simulink model "sasControl"  (R2020a)
settings: Solver=ode45  StartTime=0.0  StopTime=0.8  MaxStep=5e-06  RelTol=1e-9  AbsTol=4e-3
undefined symbols (not defined in the file): Asigma, b1, b2, bsigma, C, Csigma, CvC, Cxe, L, LiL, LoadAddResistor, LoadRemoveResistor, Masigma, Nasigma, obsControl, obsSys, P, R, Ro, SourceAddVoltage, SourceRemoveVoltage, taua1, taua2, Tmax, Vin, x0, x_e, xe
libraries: powerlib x36, PhdLibrary x8, dspsigops x3, powerlib_meascontrol x2
settings Model: SimulationMode=accelerator  Creator=d13go  LastModifiedBy=d13go
settings SolverCC: ZeroCrossControl=DisableAll  ZeroCrossAlgorithm=Adaptive
settings DebuggingCC: IgnoredZcDiagnostic=none

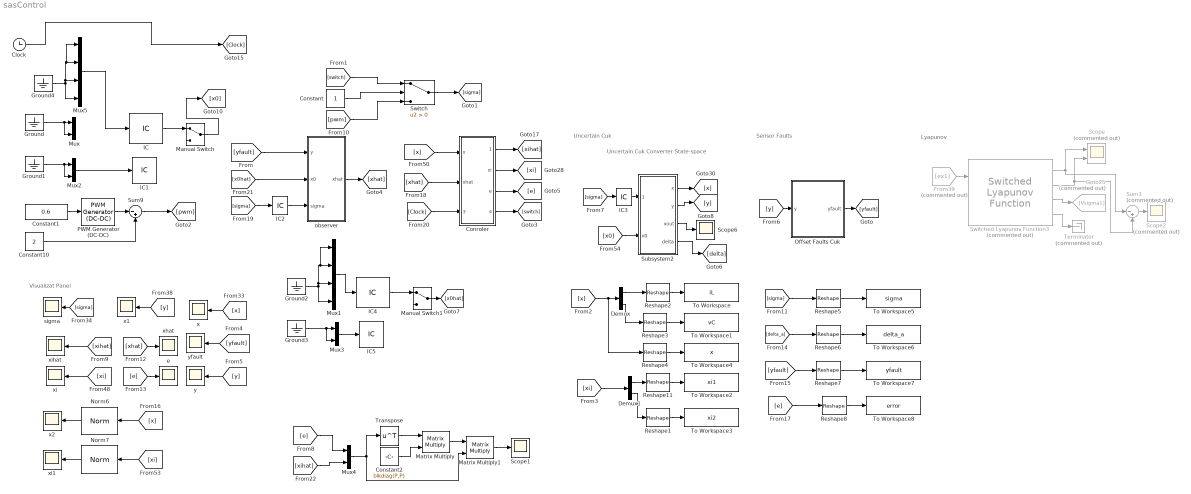
== system sasControl ==
  note: Visualizat Panel
  note: Sensor Faults
  note: Uncertain Cuk Converter
      | State-space
  note: Uncertain Cuk
  note: Lyapunov
  Clock : Clock
  Conroler : Subsystem
  Constant : Constant
  Constant1 : Constant  Value=0.6
  Constant10 : Constant  Value=2
  Constant2 : Constant  Value=blkdiag(P,P)
  Demux : Demux  Outputs=2
  Demux1 : Demux  Outputs=2
  From39 : From  Commented=on  GotoTag=ex1
  Goto25 : Goto  Commented=on  GotoTag=Vsigma1
  Ground{,1..4} (5 alike) : Ground
  IC : InitialCondition  Value=[x0]
  IC1 : InitialCondition  Value=[0 0]
  IC2 : InitialCondition  Value=2
  IC3 : InitialCondition  Value=2
  IC4 : InitialCondition  Value=[x0]
  IC5 : InitialCondition  Value=[0 0]
  Manual Switch : ManualSwitch
  Manual Switch1 : ManualSwitch
  Matrix Multiply : Product  Multiplication=Matrix(*)
  Matrix Multiply1 : Product  Multiplication=Matrix(*)
  Mux{,2..4} (4 alike) : Mux  Inputs=2
  Mux1 : Mux
  Mux5 : Mux
  Norm6 : PhdLibrary/Norms/Norm
      settings: SourceProductName=Phd Diego
  Norm7 : PhdLibrary/Norms/Norm
      settings: SourceProductName=Phd Diego
  Offset Faults Cuk : Subsystem
  PWM Generator (DC-DC) : powerlib_meascontrol/Pulse & Signal Generators/PWM Generator (DC-DC)  Fsw=10000  Ts=5e-6
  Reshape{1..8,11} (9 alike) : Reshape
  Scope : Scope  Commented=on  NumInputPorts=2
  Scope1 : Scope
  Scope2 : Scope  Commented=on
  Scope6 : Scope
  Subsystem2 : Subsystem
  Sum3 : Sum  Commented=on  Inputs=|-+
  Sum9 : Sum  Inputs=|-+
  Switch : Switch  Criteria=u2 > Threshold
  Switched Lyapunov Function3 : PhdLibrary/Switched Lyapunov Function  Commented=on  P1=obsSys{1}.lmiMat.P{1}  P2=obsSys{1}.lmiMat.P{2}
      link override Quadratic Lyapunov Function2: SourceBlock=PhdLibrary/Quadratic Lyapunov Function
      link override Quadratic Lyapunov Function3: SourceBlock=PhdLibrary/Quadratic Lyapunov Function
      settings: SourceProductName=Phd Diego
  Terminator : Terminator  Commented=on
  To Workspace : ToWorkspace  VariableName=iL  SaveFormat=Timeseries  SampleTime=-1
  To Workspace1 : ToWorkspace  VariableName=vC  SaveFormat=Timeseries  SampleTime=-1
  To Workspace2 : ToWorkspace  VariableName=xi1  SaveFormat=Timeseries  SampleTime=-1
  To Workspace3 : ToWorkspace  VariableName=xi2  SaveFormat=Timeseries  SampleTime=-1
  To Workspace4 : ToWorkspace  VariableName=x  SaveFormat=Timeseries  SampleTime=-1
  To Workspace5 : ToWorkspace  VariableName=sigma  SaveFormat=Timeseries  SampleTime=-1
  To Workspace6 : ToWorkspace  VariableName=delta_a  SaveFormat=Timeseries  SampleTime=-1
  To Workspace7 : ToWorkspace  VariableName=yfault  SaveFormat=Timeseries  SampleTime=-1
  To Workspace8 : ToWorkspace  VariableName=error  SaveFormat=Timeseries  SampleTime=-1
  Transpose : Math  Operator=transpose  SaturateOnIntegerOverflow=on
  e : Scope
  observer : Subsystem
  sigma : Scope
  x : Scope
  x1 : Scope
  x2 : Scope
  xhat : Scope
  xi : Scope
  xi1 : Scope
  xihat : Scope
  y : Scope
  yfault : Scope
  wires:
  Subsystem2/1(x) -> [x]
  Subsystem2/2(y) -> [y]
  [y] -> Offset Faults Cuk/1(y)
  Offset Faults Cuk/1(yfault) -> [yfault]
  [yfault] -> observer/1(y)
  [sigma] -> IC3/1
  [x] -> x/1
  [sigma] -> sigma/1
  [y] -> x1/1
  From39/1 -> Switched Lyapunov Function3/1
  Switched Lyapunov Function3/3 -> Goto25/1
  Switched Lyapunov Function3/4 -> Terminator/1
  Switched Lyapunov Function3/1 -> Scope/1, Sum3/1
  Switched Lyapunov Function3/2 -> Sum3/2, Scope/2
  Conroler/1(xihat) -> [xihat]
  [xihat] -> xihat/1
  [xi] -> xi/1
  Sum3/1 -> Scope2/1
  PWM Generator (DC-DC)/1 -> Sum9/1
  Constant10/1 -> Sum9/2
  Constant1/1 -> PWM Generator (DC-DC)/1
  Conroler/2(xi) -> [xi]
  [x0] -> Subsystem2/2(x0)
  Ground/1 -> Mux/2, Mux/1
  [x] -> Reshape4/1, Demux/1
  Demux/1 -> Reshape2/1
  Demux/2 -> Reshape3/1
  [xi] -> Demux1/1
  Demux1/1 -> Reshape11/1
  Reshape11/1 -> To Workspace2/1
  Reshape1/1 -> To Workspace3/1
  Demux1/2 -> Reshape1/1
  Norm7/1 -> xi1/1
  [x] -> Norm6/1
  [xi] -> Norm7/1
  Norm6/1 -> x2/1
  [yfault] -> yfault/1
  [y] -> y/1
  Ground1/1 -> Mux2/2, Mux2/1
  Mux2/1 -> IC1/1
  [x0hat] -> observer/2(x0)
  Subsystem2/3(xout) -> Scope6/1
  IC/1 -> Manual Switch/1
  Manual Switch/1 -> [x0]
  Sum9/1 -> [pwm]
  observer/1(xhat) -> [xhat]
  Conroler/3(e) -> [e]
  [xhat] -> xhat/1
  [e] -> e/1
  Reshape2/1 -> To Workspace/1
  Reshape3/1 -> To Workspace1/1
  Reshape4/1 -> To Workspace4/1
  Conroler/4(sigma) -> [switch]
  [switch] -> Switch/1
  [pwm] -> Switch/3
  Constant/1 -> Switch/2
  Switch/1 -> [sigma]
  [sigma] -> Reshape5/1
  Reshape5/1 -> To Workspace5/1
  Subsystem2/4(delta) -> [delta]
  [delta_a] -> Reshape6/1
  Reshape6/1 -> To Workspace6/1
  Reshape7/1 -> To Workspace7/1
  [yfault] -> Reshape7/1
  [e] -> Reshape8/1
  Reshape8/1 -> To Workspace8/1
  [Clock] -> Conroler/3(clock)
  [x] -> Conroler/1(x)
  [sigma] -> IC2/1
  IC2/1 -> observer/3(sigma)
  IC3/1 -> Subsystem2/1(sigma)
  [xhat] -> Conroler/2(xhat)
  Mux1/1 -> IC4/1
  Ground2/1 -> Mux1/1, Mux1/2, Mux1/3, Mux1/4
  Mux3/1 -> IC5/1
  Ground3/1 -> Mux3/2, Mux3/1
  Manual Switch1/1 -> [x0hat]
  IC4/1 -> Manual Switch1/1
  [e] -> Mux4/1
  [xihat] -> Mux4/2
  Mux4/1 -> Matrix Multiply1/2, Transpose/1
  Matrix Multiply/1 -> Matrix Multiply1/1
  Matrix Multiply1/1 -> Scope1/1
  Constant2/1 -> Matrix Multiply/2
  Transpose/1 -> Matrix Multiply/1
  Mux5/1 -> IC/1
  Ground4/1 -> Mux5/1, Mux5/2, Mux5/3, Mux5/4
  Clock/1 -> [Clock]

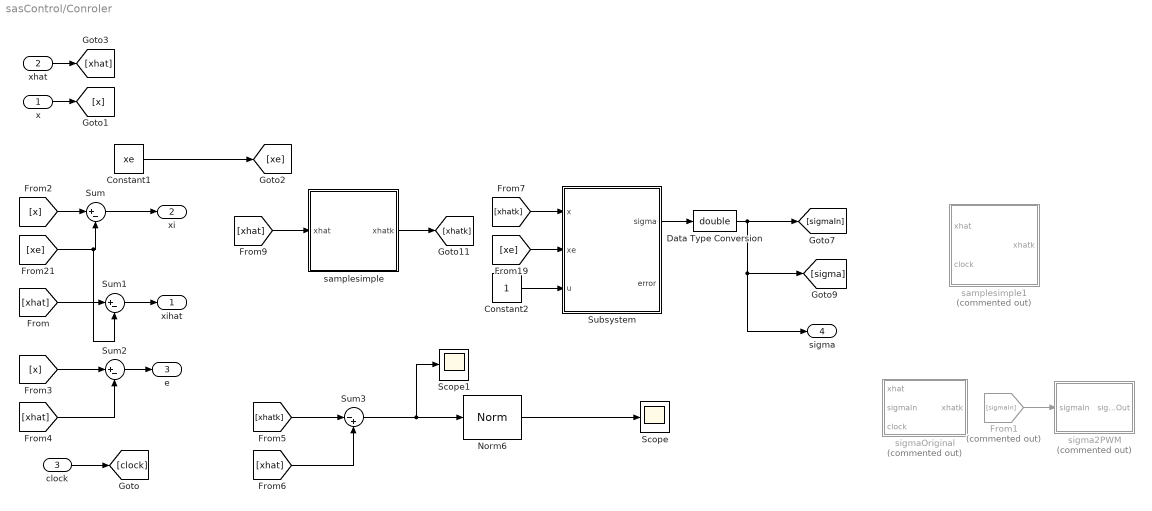
== system sasControl/Conroler ==
  x : Inport
  xhat : Inport  Port=2
  clock : Inport  Port=3
  Constant1 : Constant  Value=xe  VectorParams1D=off
  Constant2 : Constant
  Data Type Conversion : DataTypeConversion  OutDataTypeStr=double
  From1 : From  Commented=on  GotoTag=sigmaIn
  Norm6 : PhdLibrary/Norms/Norm
      settings: SourceProductName=Phd Diego
  Scope : Scope
  Scope1 : Scope
  Subsystem : Subsystem  mask{P1=obsControl.P, A1=obsControl.Asigma{1}, B1=obsControl.bsigma{1}, P2=obsControl.P, A2=obsControl.Asigma{2}, B2=obsControl.bsigma{2}}
      mask prompts: P1 "P matrx"; A1 "A matrix"; B1 "b matrix"; P2 "P matrx"; A2 "A matrix"; B2 "b matrix"
      mask DialogControl Container3 Prompt: Subsystem 1
      mask DialogControl Container3_copy Prompt: Subsystem 2
      mask Display: disp('Switching \n Control Law \n 2-Subsystems');
  Sum : Sum  Inputs=|+-
  Sum1 : Sum  Inputs=|+-
  Sum2 : Sum  Inputs=|+-
  Sum3 : Sum  Inputs=|-+
  samplesimple : Subsystem
  samplesimple1 : Subsystem  Commented=on
  sigma2PWM : Subsystem  Commented=on
  sigmaOriginal : Subsystem  Commented=on
  xihat : Outport
  xi : Outport  Port=2
  e : Outport  Port=3
  sigma : Outport  Port=4
  wires:
  [xe] -> Sum1/2, Sum/2
  xhat/1 -> [xhat]
  x/1 -> [x]
  Sum2/1 -> e/1
  samplesimple/1("xhatk ") -> [xhatk]
  Sum1/1 -> xihat/1
  [xe] -> Subsystem/2(xe)
  Constant2/1 -> Subsystem/3(u)
  Subsystem/1(sigma) -> Data Type Conversion/1
  Data Type Conversion/1 -> sigma/1, [sigma], [sigmaIn]
  From1/1 -> sigma2PWM/1(sigmaIn)
  clock/1 -> [clock]
  Sum/1 -> xi/1
  Constant1/1 -> [xe]
  [xhat] -> Sum1/1
  [x] -> Sum/1
  [x] -> Sum2/1
  [xhat] -> Sum2/2
  [xhatk] -> Sum3/1
  Sum3/1 -> Scope1/1, Norm6/1
  [xhat] -> Sum3/2
  Norm6/1 -> Scope/1
  [xhat] -> samplesimple/1(xhat)
  [xhatk] -> Subsystem/1(x)

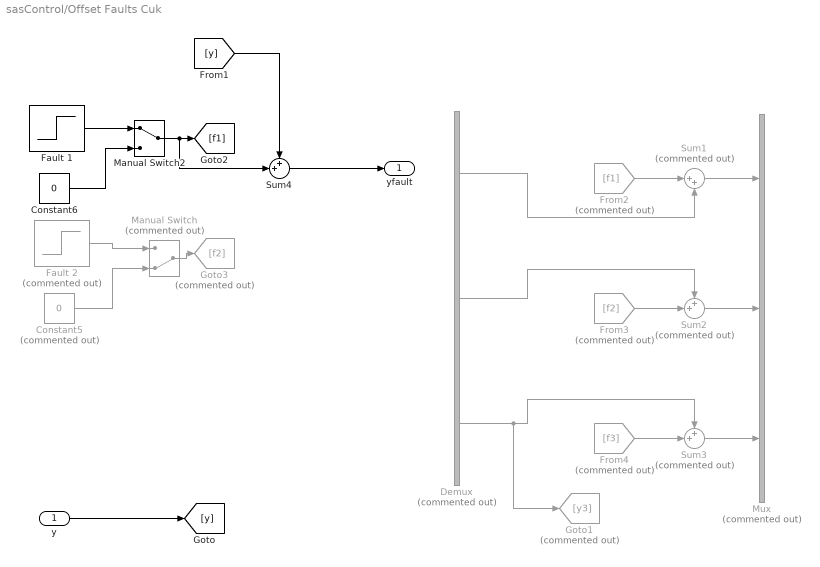
== system sasControl/Offset Faults Cuk ==
  y : Inport
  Constant5 : Constant  Commented=on  Value=0
  Constant6 : Constant  Value=0
  Demux : Demux  Commented=on  Outputs=3
  Fault 1 : Step  Time=0.35  After=0.5/7*Cxe(1)  SampleTime=0
  Fault 2 : Step  Commented=on  Time=0.35  After=0.075*Cxe(2)  SampleTime=0
  From2 : From  Commented=on  GotoTag=f1
  From3 : From  Commented=on  GotoTag=f2
  From4 : From  Commented=on  GotoTag=f3
  Goto1 : Goto  Commented=on  GotoTag=y3
  Goto3 : Goto  Commented=on  GotoTag=f2
  Manual Switch : ManualSwitch  Commented=on  CurrentSetting=0
  Manual Switch2 : ManualSwitch
  Mux : Mux  Commented=on  Inputs=3
  Sum1 : Sum  Commented=on  Inputs=|++
  Sum2 : Sum  Commented=on  Inputs=++|
  Sum3 : Sum  Commented=on  Inputs=++|
  Sum4 : Sum  Inputs=++|
  yfault : Outport
  wires:
  Fault 2/1 -> Manual Switch/1
  Fault 1/1 -> Manual Switch2/1
  Constant5/1 -> Manual Switch/2
  Constant6/1 -> Manual Switch2/2
  Sum1/1 -> Mux/1
  Sum3/1 -> Mux/3
  y/1 -> [y]
  Sum2/1 -> Mux/2
  Manual Switch2/1 -> Sum4/2, [f1]
  From2/1 -> Sum1/1
  Manual Switch/1 -> Goto3/1
  From3/1 -> Sum2/2
  From4/1 -> Sum3/2
  Demux/1 -> Sum1/2
  Demux/2 -> Sum2/1
  Demux/3 -> Goto1/1, Sum3/1
  [y] -> Sum4/1
  Sum4/1 -> yfault/1

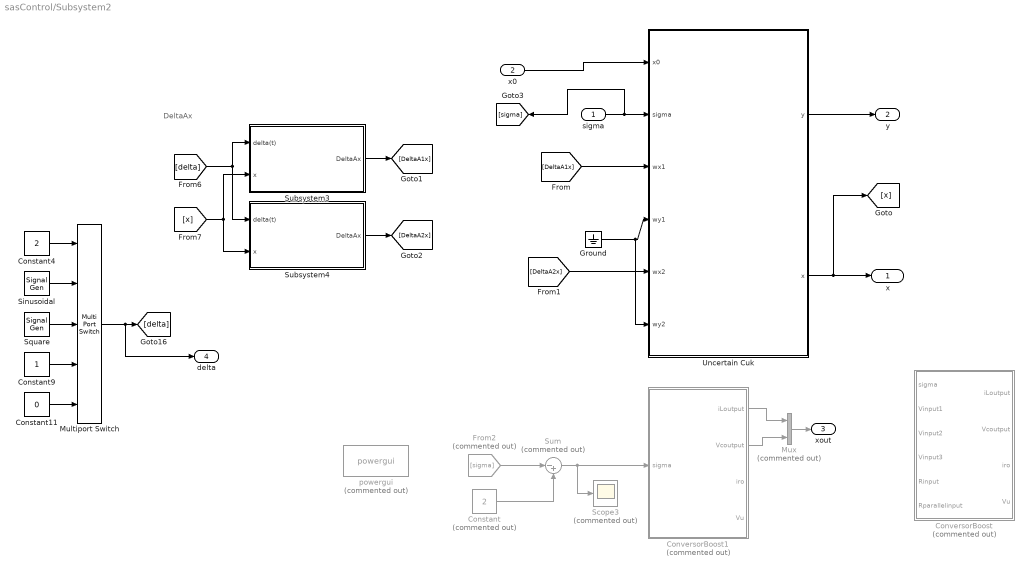
== system sasControl/Subsystem2 ==
  note: DeltaAx
  sigma : Inport
  x0 : Inport  Port=2
  Constant : Constant  Commented=on  Value=2
  Constant11 : Constant  Value=0
  Constant4 : Constant  Value=2
  Constant9 : Constant
  ConversorBoost : Subsystem  Commented=on
  ConversorBoost1 : Subsystem  Commented=on
  From2 : From  Commented=on  GotoTag=sigma
  Ground : Ground
  Multiport Switch : MultiPortSwitch  Inputs=4
  Mux : Mux  Commented=on  Inputs=2
  Scope3 : Scope  Commented=on
  Sinusoidal : SignalGenerator  Amplitude=20  Frequency=60  Units=rad/sec
  Square : SignalGenerator  WaveForm=square  Frequency=300  Units=rad/sec
  Subsystem3 : Subsystem  mask{M=Masigma{1}, N=Nasigma{1}}
      mask prompts: M "M matrix"; N "N matrix"
      mask DialogControl DescTextVar Prompt: Uncertainties matrices of type \DeltaA = delta(t)*MaNa*x(t)
      mask Display: disp('Norm-bounded \n uncertainty')
  Subsystem4 : Subsystem  mask{M=Masigma{2}, N=Nasigma{2}}
      mask prompts: M "M matrix"; N "N matrix"
      mask DialogControl DescTextVar Prompt: Uncertainties matrices of type \DeltaA = delta(t)*MaNa*x(t)
      mask Display: disp('Norm-bounded \n uncertainty')
  Sum : Sum  Commented=on  Inputs=|-+
  Uncertain Cuk : Subsystem  mask{A1=Asigma{1}, B1=bsigma{1}, C1=Csigma{1}, A2=Asigma{2}, B2=bsigma{2}, C2=Csigma{2}}
      mask prompts: A1 "Matrix A"; B1 "Matrix B"; C1 "Matrix C"; A2 "Matrix A"; B2 "Matrix B"; C2 "Matrix C"
      mask DialogControl DescTextVar Prompt: dx/dt = A(sigma)x+ B(sigma)u + wx(sigma,x,u,t)
      mask DialogControl Control2 Prompt: y = C(sigma)x + wy(sigma,x,u,t)
      mask DialogControl Container3 Prompt: Subsystem 1
      mask DialogControl Container4 Prompt: Subsystem 2
      mask Display: disp('Switched Perturbed State Space \n 2-Subsystems')
  powergui : powerlib/powergui  Priority=1  Commented=on  SimulationMode=Continuous  SampleTime=50e-6  frequency=60  Iterations=50  frequencyindice=0  Pbase=100e6  ErrMax=1e-4  UnitsV=kV  UnitsW=MW  buscounter=0  FunctionMessages=off  echomessages=off  EnableUseOfTLC=off  CurrentSourceSwitches=off  DisableSnubberDevices=off  DisableRonSwitches=off  DisableVfSwitches=off  DisplayEquations=off  AutomaticDiscreteSolvers=off  SolverType=Tustin/Backward Euler (TBE)  Interpol=off  ExternalGateDelay=off  methode=off  Ts=100  x0status=blocks  SPID=on  SwTol=0  HookPort=off  NonlinearTolerance=1e-4  nMaxIteration=100  ContinueOnMaxIteration=off  RestoreLinks=warning  ResistiveCurrentMeasurement=off  Frange=[0:2:500]  Ylog=off  Xlog=on  ShowGrid=off  save=off  variable=ZData  structure=0  ZoomFFT=off  StartTime=0.0  cycles=1  DisplayStyle=1  fundamental=60  FreqAxis=off  MaxFrequency=1000  frequencyindicesteady=1  RmsSteady=1  display=off
  x : Outport
  y : Outport  Port=2
  xout : Outport  Port=3
  delta : Outport  Port=4
  wires:
  x0/1 -> Uncertain Cuk/1(x0)
  Uncertain Cuk/2(x) -> [x], x/1
  Uncertain Cuk/1(y) -> y/1
  sigma/1 -> [sigma], Uncertain Cuk/2(sigma)
  [DeltaA1x] -> Uncertain Cuk/3(wx1)
  Constant9/1 -> Multiport Switch/4
  Sinusoidal/1 -> Multiport Switch/2
  Constant4/1 -> Multiport Switch/1
  Square/1 -> Multiport Switch/3
  Constant11/1 -> Multiport Switch/5
  [DeltaA2x] -> Uncertain Cuk/5(wx2)
  Multiport Switch/1 -> delta/1, [delta]
  Subsystem3/1(DeltaAx) -> [DeltaA1x]
  [x] -> Subsystem4/2(x), Subsystem3/2(x)
  [delta] -> Subsystem3/1(delta(t)), Subsystem4/1(delta(t))
  Ground/1 -> Uncertain Cuk/6(wy2), Uncertain Cuk/4(wy1)
  Subsystem4/1(DeltaAx) -> [DeltaA2x]
  ConversorBoost1/1(iLoutput) -> Mux/1
  ConversorBoost1/2(Vcoutput) -> Mux/2
  Mux/1 -> xout/1
  From2/1 -> Sum/1
  Sum/1 -> Scope3/1, ConversorBoost1/1(sigma)
  Constant/1 -> Sum/2

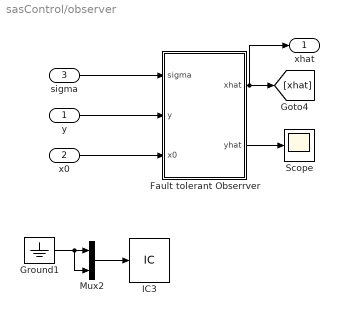
== system sasControl/observer ==
  y : Inport
  x0 : Inport  Port=2
  sigma : Inport  Port=3
  Fault tolerant Obserrver : Subsystem  mask(Boots State-Space model){A1=obsControl.Asigma{1,1}, A2=obsControl.Asigma{1,2}, B1=obsControl.bsigma{1,1}, Cmatrix=obsControl.Csigma{1,1}, L1=10*obsControl.Lcsigma{1,1}, L2=10*obsControl.Lcsigma{1,2}}
      mask prompts: A1 "A1 matrix"; A2 "A2 matrix"; B1 "B matrix"; Cmatrix "Output Matrix"; L1 "L1 matrix"; L2 "L2 matrix"
      mask help: Boots State-Space model
      mask Display: disp('Observer')
  Ground1 : Ground
  IC3 : InitialCondition  Value=[51 151]
  Mux2 : Mux  Inputs=2
  Scope : Scope
  xhat : Outport
  wires:
  Fault tolerant Obserrver/2(yhat) -> Scope/1
  y/1 -> Fault tolerant Obserrver/2(y)
  Fault tolerant Obserrver/1(xhat) -> xhat/1, [xhat]
  sigma/1 -> Fault tolerant Obserrver/1(sigma)
  Ground1/1 -> Mux2/2, Mux2/1
  Mux2/1 -> IC3/1
  x0/1 -> Fault tolerant Obserrver/3(x0)

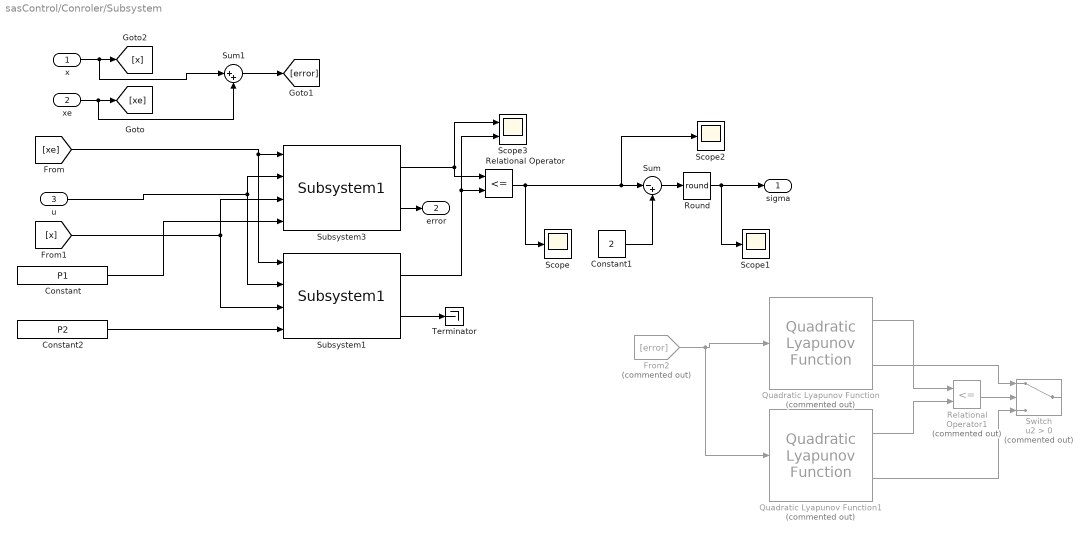
== system sasControl/Conroler/Subsystem ==
  x : Inport
  xe : Inport  Port=2
  u : Inport  Port=3
  Constant : Constant  Value=P1
  Constant1 : Constant  Value=2
  Constant2 : Constant  Value=P2
  From2 : From  Commented=on  GotoTag=error
  Quadratic Lyapunov Function : PhdLibrary/Quadratic Lyapunov Function  Commented=on  P=P1
      settings: SourceProductName=Phd Diego
  Quadratic Lyapunov Function1 : PhdLibrary/Quadratic Lyapunov Function  Commented=on  P=P2
      settings: SourceProductName=Phd Diego
  Relational Operator : RelationalOperator  Operator=<=  OutDataTypeStr=boolean  RndMeth=Nearest
  Relational Operator1 : RelationalOperator  Commented=on  Operator=<=  OutDataTypeStr=boolean  RndMeth=Nearest
  Round : Rounding  Operator=round
  Scope : Scope
  Scope1 : Scope
  Scope2 : Scope
  Scope3 : Scope  NumInputPorts=2
  Subsystem1 : PhdLibrary/Controllers/Subsystem1  A=A2  B=B2
      settings: SourceProductName=Phd Diego
  Subsystem3 : PhdLibrary/Controllers/Subsystem1  A=A1  B=B1
      settings: SourceProductName=Phd Diego
  Sum : Sum  Inputs=|-+
  Sum1 : Sum  Inputs=|++
  Switch : Switch  Commented=on  Criteria=u2 > Threshold
  Terminator : Terminator
  sigma : Outport
  error : Outport  Port=2
  wires:
  x/1 -> Sum1/1, [x]
  [xe] -> Subsystem1/1, Subsystem3/1
  [x] -> Subsystem1/3, Subsystem3/3
  u/1 -> Subsystem1/2, Subsystem3/2
  Subsystem1/2 -> Terminator/1
  Subsystem3/2 -> error/1
  Subsystem1/1 -> Scope3/2, Relational Operator/2
  Subsystem3/1 -> Relational Operator/1, Scope3/1
  Relational Operator/1 -> Scope2/1, Sum/1, Scope/1
  Constant1/1 -> Sum/2
  Sum/1 -> Round/1
  Round/1 -> Scope1/1, sigma/1
  xe/1 -> [xe], Sum1/2
  Sum1/1 -> [error]
  From2/1 -> Quadratic Lyapunov Function1/1, Quadratic Lyapunov Function/1
  Quadratic Lyapunov Function1/1 -> Relational Operator1/2
  Relational Operator1/1 -> Switch/2
  Quadratic Lyapunov Function1/2 -> Switch/3
  Quadratic Lyapunov Function/1 -> Relational Operator1/1
  Quadratic Lyapunov Function/2 -> Switch/1
  Constant/1 -> Subsystem3/4
  Constant2/1 -> Subsystem1/4

== system sasControl/Conroler/samplesimple ==
  xhat : Inport
  NOT : Logic  Operator=NOT  IconShape=distinctive  AllPortsSameDT=off  OutDataTypeStr=boolean
  Pulse Generator : DiscretePulseGenerator  PulseType=Time based  Period=2*10e-6  PulseWidth=50
  Sample and Hold : dspsigops/Sample and Hold  trig=Either edge  initCond=1  latchinput=off
  Scope : Scope
  "xhatk " : Outport
  wires:
  xhat/1 -> Sample and Hold/1
  Sample and Hold/1 -> Scope/1, "xhatk "/1
  Pulse Generator/1 -> NOT/1
  NOT/1 -> Sample and Hold/Trigger

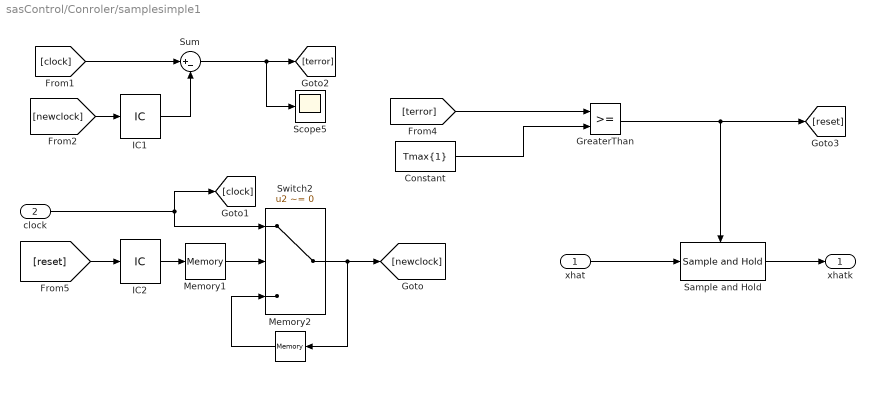
== system sasControl/Conroler/samplesimple1 ==
  xhat : Inport
  clock : Inport  Port=2
  Constant : Constant  Value=Tmax{1}
  GreaterThan : RelationalOperator  OutDataTypeStr=boolean  RndMeth=Simplest
  IC1 : InitialCondition  Value=0
  IC2 : InitialCondition  Value=0
  Memory1 : Memory  InheritSampleTime=on
  Memory2 : Memory  InheritSampleTime=on
  Sample and Hold : dspsigops/Sample and Hold  trig=Rising edge  initCond=1  latchinput=off
  Scope5 : Scope
  Sum : Sum  Inputs=|+-
  Switch2 : Switch  Criteria=u2 ~= 0
  "xhatk " : Outport
  wires:
  xhat/1 -> Sample and Hold/1
  Sample and Hold/1 -> "xhatk "/1
  [clock] -> Sum/1
  Sum/1 -> Scope5/1, [terror]
  Constant/1 -> GreaterThan/2
  [terror] -> GreaterThan/1
  GreaterThan/1 -> [reset], Sample and Hold/Trigger
  clock/1 -> [clock], Switch2/1
  [newclock] -> IC1/1
  IC1/1 -> Sum/2
  Switch2/1 -> [newclock], Memory2/1
  Memory2/1 -> Switch2/3
  [reset] -> IC2/1
  Memory1/1 -> Switch2/2
  IC2/1 -> Memory1/1

== system sasControl/Conroler/sigma2PWM ==
  sigmaIn : Inport
  Constant1 : Constant
  Constant10 : Constant  Value=2
  Constant3 : Constant  Value=0
  PWM Generator (DC-DC) : powerlib_meascontrol/Pulse & Signal Generators/PWM Generator (DC-DC)  Fsw=1  Ts=5e-6
  Sum9 : Sum  Inputs=|-+
  Switch1 : Switch  Threshold=2
  sigmaOut : Outport
  wires:
  Switch1/1 -> PWM Generator (DC-DC)/1
  PWM Generator (DC-DC)/1 -> Sum9/1
  Constant3/1 -> Switch1/1
  sigmaIn/1 -> Switch1/2
  Constant10/1 -> Sum9/2
  Sum9/1 -> sigmaOut/1
  Constant1/1 -> Switch1/3

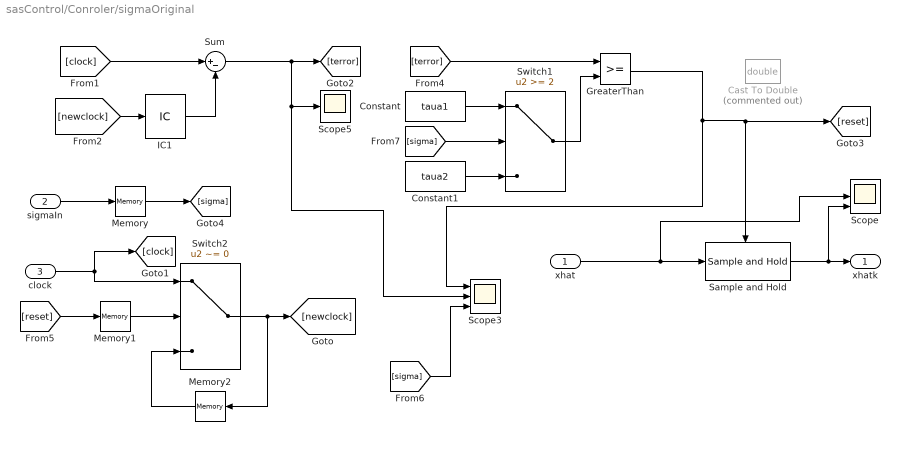
== system sasControl/Conroler/sigmaOriginal ==
  xhat : Inport
  sigmaIn : Inport  Port=2
  clock : Inport  Port=3
  Cast To Double : DataTypeConversion  Commented=on  OutDataTypeStr=double
  Constant : Constant  Value=taua1
  Constant1 : Constant  Value=taua2
  GreaterThan : RelationalOperator  OutDataTypeStr=boolean  RndMeth=Simplest
  IC1 : InitialCondition  Value=0
  Memory : Memory  InitialCondition=2  InheritSampleTime=on
  Memory1 : Memory  InitialCondition=2  InheritSampleTime=on
  Memory2 : Memory  InheritSampleTime=on
  Sample and Hold : dspsigops/Sample and Hold  trig=Rising edge  initCond=1  latchinput=off
  Scope : Scope  NumInputPorts=3
  Scope3 : Scope  NumInputPorts=3
  Scope5 : Scope
  Sum : Sum  Inputs=|+-
  Switch1 : Switch  Threshold=2
  Switch2 : Switch  Criteria=u2 ~= 0
  "xhatk " : Outport
  wires:
  xhat/1 -> Scope/2, Sample and Hold/1
  Sample and Hold/1 -> Scope/3, "xhatk "/1
  [clock] -> Sum/1
  Sum/1 -> Scope3/2, Scope5/1, [terror]
  Constant/1 -> Switch1/1
  Constant1/1 -> Switch1/3
  [terror] -> GreaterThan/1
  Switch1/1 -> GreaterThan/2
  GreaterThan/1 -> [reset], Sample and Hold/Trigger, Scope3/1
  clock/1 -> [clock], Switch2/1
  [reset] -> Memory1/1
  Memory1/1 -> Switch2/2
  [newclock] -> IC1/1
  IC1/1 -> Sum/2
  [sigma] -> Scope3/3
  Switch2/1 -> Memory2/1, [newclock]
  Memory2/1 -> Switch2/3
  [sigma] -> Switch1/2
  sigmaIn/1 -> Memory/1
  Memory/1 -> [sigma]

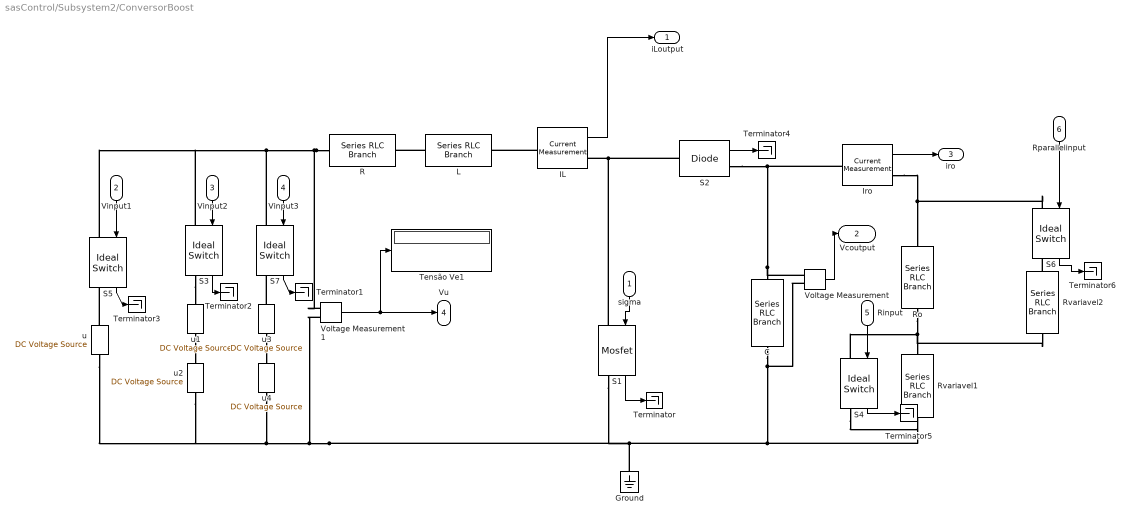
== system sasControl/Subsystem2/ConversorBoost ==
  sigma : Inport
  Vinput1 : Inport  Port=2
  Vinput2 : Inport  Port=3
  Vinput3 : Inport  Port=4
  Rinput : Inport  Port=5
  Rparallelinput : Inport  Port=6
  C : powerlib/Elements/Series RLC Branch  LConnTagsString=__new0  RConnTagsString=__new0  BranchType=C  Resistance=1  Inductance=1e-3  SetiL0=off  InitialCurrent=0  Capacitance=C  Setx0=on  InitialVoltage=0  Measurements=None
  Ground : powerlib/Elements/Ground  LConnTagsString=a
  IL : powerlib/Measurements/Current Measurement  PhasorSimulation=off  OutputType=Complex  PSBequivalent=0
  Iro : powerlib/Measurements/Current Measurement  PhasorSimulation=off  OutputType=Complex  PSBequivalent=0
  L : powerlib/Elements/Series RLC Branch  LConnTagsString=__new0  RConnTagsString=__new0  BranchType=L  Resistance=1  Inductance=L  SetiL0=on  InitialCurrent=0  Capacitance=1e-6  Setx0=off  InitialVoltage=0  Measurements=None
  R : powerlib/Elements/Series RLC Branch  LConnTagsString=__new0  RConnTagsString=__new0  BranchType=R  Resistance=R  Inductance=1e-3  SetiL0=off  InitialCurrent=0  Capacitance=1e-6  Setx0=off  InitialVoltage=0  Measurements=None
  Ro : powerlib/Elements/Series RLC Branch  LConnTagsString=__new0  RConnTagsString=__new0  BranchType=R  Resistance=Ro  Inductance=1e-3  SetiL0=off  InitialCurrent=0  Capacitance=1e-6  Setx0=off  InitialVoltage=0  Measurements=None
  Rvariavel1 : powerlib/Elements/Series RLC Branch  LConnTagsString=__new0  RConnTagsString=__new0  BranchType=R  Resistance=LoadAddResistor  Inductance=1e-3  SetiL0=off  InitialCurrent=0  Capacitance=1e-6  Setx0=off  InitialVoltage=0  Measurements=None
  Rvariavel2 : powerlib/Elements/Series RLC Branch  LConnTagsString=__new0  RConnTagsString=__new0  BranchType=R  Resistance=LoadRemoveResistor  Inductance=1e-3  SetiL0=off  InitialCurrent=0  Capacitance=1e-6  Setx0=off  InitialVoltage=0  Measurements=None
  S1 : powerlib/Power Electronics/Mosfet  Ron=0.0000001  Lon=0  Rd=0.000000001  Vfd=0  IC=0  Rs=1e5  Cs=inf  Measurements=on
  S2 : powerlib/Power Electronics/Diode  Ron=0.000001  Lon=0  Vf=0  IC=0  UseSnubber=off  Rs=0  Cs=0  Measurements=on
  S{3..7} (5 alike) : powerlib/Power Electronics/Ideal Switch  Ron=0.0000001  Lon=0  IC=0  Rs=1e8  Cs=inf  Measurements=on
  Tensão Ve1 : Display
  Terminator{,1..6} (7 alike) : Terminator
  Voltage Measurement : powerlib/Measurements/Voltage Measurement  PhasorSimulation=off  OutputType=Complex  PSBequivalent=0
  Voltage Measurement1 : powerlib/Measurements/Voltage Measurement  PhasorSimulation=off  OutputType=Complex  PSBequivalent=0
  u : powerlib/Electrical Sources/DC Voltage Source  Amplitude=u  Measurements=None
  u1 : powerlib/Electrical Sources/DC Voltage Source  Amplitude=SourceAddVoltage  Measurements=None
  u2 : powerlib/Electrical Sources/DC Voltage Source  Amplitude=u  Measurements=None
  u3 : powerlib/Electrical Sources/DC Voltage Source  Amplitude=SourceRemoveVoltage  Measurements=None
  u4 : powerlib/Electrical Sources/DC Voltage Source  Amplitude=u  Measurements=None
  iLoutput : Outport
  Vcoutput : Outport  Port=2
  iro : Outport  Port=3
  Vu : Outport  Port=4
  wires:
  Rinput/1 -> S4/1
  IL/1 -> iLoutput/1
  sigma/1 -> S1/1
  Voltage Measurement/1 -> Vcoutput/1
  Iro/1 -> iro/1
  Voltage Measurement1/1 -> Vu/1, Tensão Ve1/1
  Vinput1/1 -> S5/1
  Vinput2/1 -> S3/1
  Rparallelinput/1 -> S6/1
  Vinput3/1 -> S7/1
  S1/1 -> Terminator/1
  S7/1 -> Terminator1/1
  S3/1 -> Terminator2/1
  S5/1 -> Terminator3/1
  S2/1 -> Terminator4/1
  S4/1 -> Terminator5/1
  S6/1 -> Terminator6/1
  connections:
  Ro/RConn1 -- Rvariavel2/LConn1 -- Rvariavel1/RConn1 -- S4/LConn1
  IL/LConn1 -- L/RConn1
  C/RConn1 -- S4/RConn1 -- Rvariavel1/LConn1 -- S1/RConn1 -- u2/LConn1 -- u/LConn1 -- u4/LConn1 -- Voltage Measurement1/LConn2 -- Ground/LConn1 -- Voltage Measurement/LConn2
  S2/LConn1 -- S1/LConn1 -- IL/RConn1
  R/LConn1 -- S3/LConn1 -- S5/LConn1 -- S7/LConn1 -- Voltage Measurement1/LConn1
  Iro/RConn1 -- S6/LConn1 -- Ro/LConn1
  L/LConn1 -- R/RConn1
  S2/RConn1 -- Iro/LConn1 -- Voltage Measurement/LConn1 -- C/LConn1
  u/RConn1 -- S5/RConn1
  Rvariavel2/RConn1 -- S6/RConn1
  S3/RConn1 -- u1/RConn1
  u1/LConn1 -- u2/RConn1
  u3/LConn1 -- S7/RConn1
  u3/RConn1 -- u4/RConn1

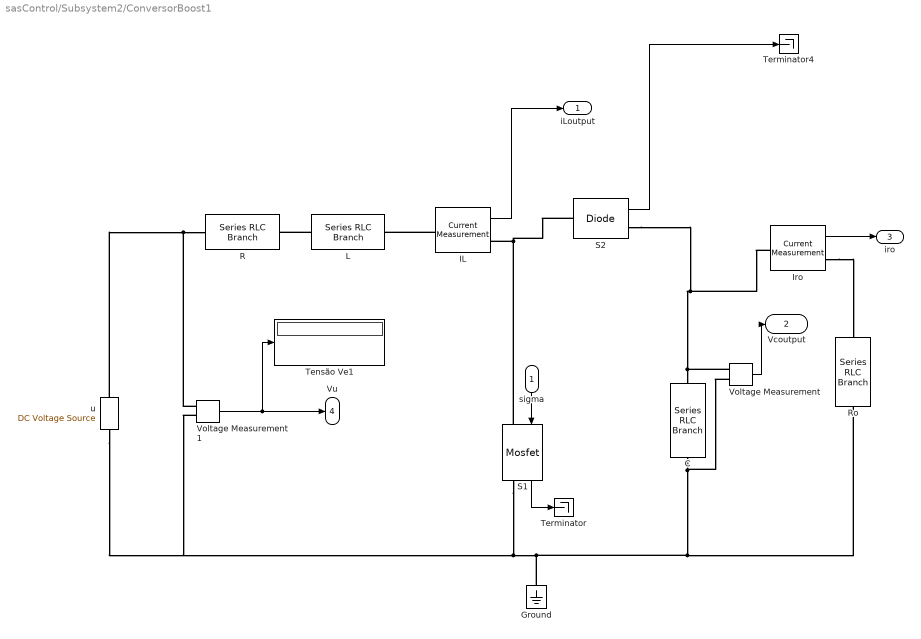
== system sasControl/Subsystem2/ConversorBoost1 ==
  sigma : Inport
  C : powerlib/Elements/Series RLC Branch  LConnTagsString=__new0  RConnTagsString=__new0  BranchType=C  Resistance=1  Inductance=1e-3  SetiL0=off  InitialCurrent=0  Capacitance=CvC  Setx0=on  InitialVoltage=xe(2)  Measurements=None
  Ground : powerlib/Elements/Ground  LConnTagsString=a
  IL : powerlib/Measurements/Current Measurement  PhasorSimulation=off  OutputType=Complex  PSBequivalent=0
  Iro : powerlib/Measurements/Current Measurement  PhasorSimulation=off  OutputType=Complex  PSBequivalent=0
  L : powerlib/Elements/Series RLC Branch  LConnTagsString=__new0  RConnTagsString=__new0  BranchType=L  Resistance=1  Inductance=LiL  SetiL0=on  InitialCurrent=0  Capacitance=1e-6  Setx0=off  InitialVoltage=0  Measurements=None
  R : powerlib/Elements/Series RLC Branch  LConnTagsString=__new0  RConnTagsString=__new0  BranchType=R  Resistance=R  Inductance=1e-3  SetiL0=off  InitialCurrent=0  Capacitance=1e-6  Setx0=off  InitialVoltage=0  Measurements=None
  Ro : powerlib/Elements/Series RLC Branch  LConnTagsString=__new0  RConnTagsString=__new0  BranchType=R  Resistance=Ro  Inductance=1e-3  SetiL0=off  InitialCurrent=0  Capacitance=1e-6  Setx0=off  InitialVoltage=0  Measurements=None
  S1 : powerlib/Power Electronics/Mosfet  Ron=0.0000001  Lon=0  Rd=0.000000001  Vfd=0  IC=0  Rs=1e5  Cs=inf  Measurements=on
  S2 : powerlib/Power Electronics/Diode  Ron=0.000001  Lon=0  Vf=0  IC=0  UseSnubber=off  Rs=0  Cs=0  Measurements=on
  Tensão Ve1 : Display
  Terminator : Terminator
  Terminator4 : Terminator
  Voltage Measurement : powerlib/Measurements/Voltage Measurement  PhasorSimulation=off  OutputType=Complex  PSBequivalent=0
  Voltage Measurement1 : powerlib/Measurements/Voltage Measurement  PhasorSimulation=off  OutputType=Complex  PSBequivalent=0
  u : powerlib/Electrical Sources/DC Voltage Source  Amplitude=Vin  Measurements=None
  iLoutput : Outport
  Vcoutput : Outport  Port=2
  iro : Outport  Port=3
  Vu : Outport  Port=4
  wires:
  IL/1 -> iLoutput/1
  sigma/1 -> S1/1
  Voltage Measurement/1 -> Vcoutput/1
  Iro/1 -> iro/1
  Voltage Measurement1/1 -> Vu/1, Tensão Ve1/1
  S1/1 -> Terminator/1
  S2/1 -> Terminator4/1
  connections:
  C/RConn1 -- Voltage Measurement/LConn2 -- Ro/RConn1 -- u/LConn1 -- Voltage Measurement1/LConn2 -- S1/RConn1 -- Ground/LConn1
  IL/LConn1 -- L/RConn1
  Voltage Measurement1/LConn1 -- u/RConn1 -- R/LConn1
  Iro/RConn1 -- Ro/LConn1
  L/LConn1 -- R/RConn1
  Iro/LConn1 -- S2/RConn1 -- Voltage Measurement/LConn1 -- C/LConn1
  S1/LConn1 -- S2/LConn1 -- IL/RConn1

== system sasControl/Subsystem2/Subsystem3 ==
  delta(t) : Inport
  x : Inport  Port=2
  Constant : Constant  Value=M
  Constant1 : Constant  Value=N
  Matrix Multiply1 : Product
  Matrix Multiply2 : Product  Multiplication=Matrix(*)
  Matrix Multiply3 : Product  Multiplication=Matrix(*)
  DeltaAx : Outport
  wires:
  Constant/1 -> Matrix Multiply3/1
  Constant1/1 -> Matrix Multiply3/2
  Matrix Multiply3/1 -> Matrix Multiply1/2
  delta(t)/1 -> Matrix Multiply1/1
  Matrix Multiply1/1 -> Matrix Multiply2/1
  x/1 -> Matrix Multiply2/2
  Matrix Multiply2/1 -> DeltaAx/1

== system sasControl/Subsystem2/Subsystem4 ==
  delta(t) : Inport
  x : Inport  Port=2
  Constant : Constant  Value=M
  Constant1 : Constant  Value=N
  Matrix Multiply1 : Product
  Matrix Multiply2 : Product  Multiplication=Matrix(*)
  Matrix Multiply3 : Product  Multiplication=Matrix(*)
  DeltaAx : Outport
  wires:
  Constant/1 -> Matrix Multiply3/1
  Constant1/1 -> Matrix Multiply3/2
  Matrix Multiply3/1 -> Matrix Multiply1/2
  delta(t)/1 -> Matrix Multiply1/1
  Matrix Multiply1/1 -> Matrix Multiply2/1
  x/1 -> Matrix Multiply2/2
  Matrix Multiply2/1 -> DeltaAx/1

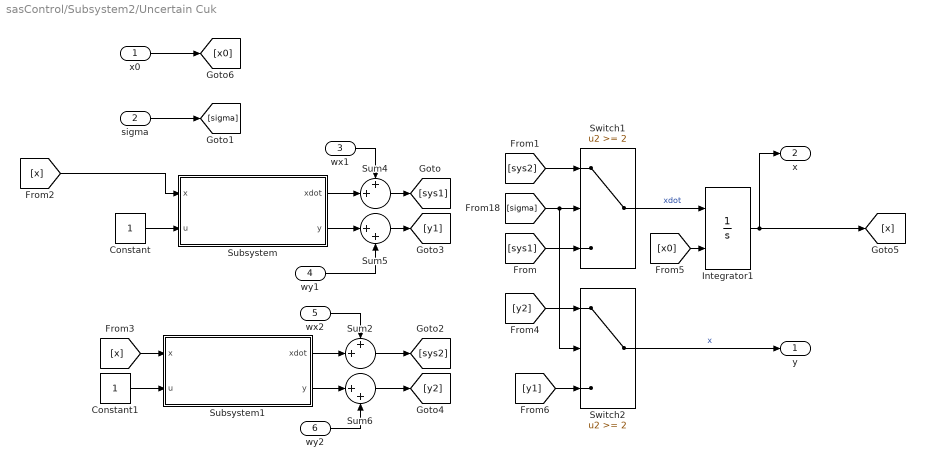
== system sasControl/Subsystem2/Uncertain Cuk ==
  x0 : Inport
  sigma : Inport  Port=2
  wx1 : Inport  Port=3
  wy1 : Inport  Port=4
  wx2 : Inport  Port=5
  wy2 : Inport  Port=6
  Constant : Constant
  Constant1 : Constant
  Integrator1 : Integrator  InitialConditionSource=external  InitialCondition=[-x_e; 0; 0]
  Subsystem : Subsystem  mask{A=A1, B=B1, C=C1}
      mask prompts: A "Matrix A"; B "Matrix B"; C "Matrix C"
      mask Display: disp('Static State Space \n xdot = Ax+Bu\n y =Cx')
  Subsystem1 : Subsystem  mask{A=A2, B=B2, C=C2}
      mask prompts: A "Matrix A"; B "Matrix B"; C "Matrix C"
      mask Display: disp('Static State Space \n xdot = Ax+Bu\n y =Cx')
  Sum2 : Sum  Inputs=++|
  Sum4 : Sum  Inputs=++|
  Sum5 : Sum  Inputs=|++
  Sum6 : Sum  Inputs=|++
  Switch1 : Switch  Threshold=2
  Switch2 : Switch  Threshold=2
  y : Outport
  x : Outport  Port=2
  wires:
  [sys2] -> Switch1/1
  [sys1] -> Switch1/3
  [sigma] -> Switch2/2, Switch1/2
  Subsystem/1(xdot) -> Sum4/2
  Subsystem/2(y) -> Sum5/1
  Sum4/1 -> [sys1]
  Sum5/1 -> [y1]
  Constant/1 -> Subsystem/2(u)
  Switch1/1 -> Integrator1/1  "xdot"
  [x0] -> Integrator1/2
  Sum6/1 -> [y2]
  Sum2/1 -> [sys2]
  Subsystem1/2(y) -> Sum6/1
  [x] -> Subsystem1/1(x)
  Subsystem1/1(xdot) -> Sum2/2
  Constant1/1 -> Subsystem1/2(u)
  [y2] -> Switch2/1
  [y1] -> Switch2/3
  Switch2/1 -> y/1  "x"
  sigma/1 -> [sigma]
  x0/1 -> [x0]
  wx1/1 -> Sum4/1
  wy1/1 -> Sum5/2
  wx2/1 -> Sum2/1
  wy2/1 -> Sum6/2
  [x] -> Subsystem/1(x)
  Integrator1/1 -> x/1, [x]

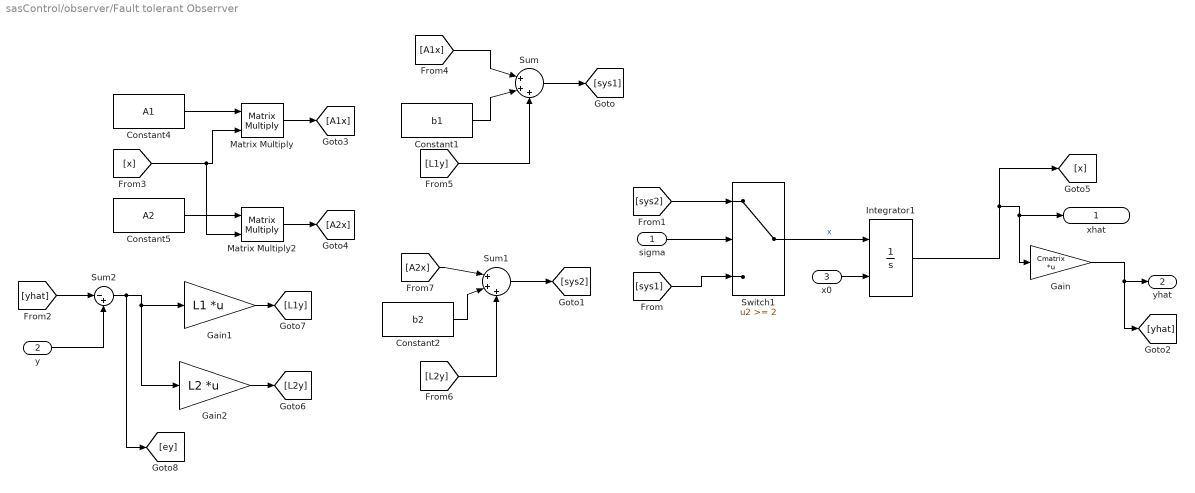
== system sasControl/observer/Fault tolerant Obserrver ==
  sigma : Inport
  y : Inport  Port=2
  x0 : Inport  Port=3
  Constant1 : Constant  Value=b1  VectorParams1D=off
  Constant2 : Constant  Value=b2  VectorParams1D=off
  Constant4 : Constant  Value=A1  VectorParams1D=off
  Constant5 : Constant  Value=A2  VectorParams1D=off
  Gain : Gain  Gain=Cmatrix  Multiplication=Matrix(K*u)
  Gain1 : Gain  Gain=L1  Multiplication=Matrix(K*u) (u vector)
  Gain2 : Gain  Gain=L2  Multiplication=Matrix(K*u) (u vector)
  Integrator1 : Integrator  InitialConditionSource=external  InitialCondition=[-x_e; 0; 0]
  Matrix Multiply : Product  Multiplication=Matrix(*)
  Matrix Multiply2 : Product  Multiplication=Matrix(*)
  Sum : Sum  Inputs=|+++
  Sum1 : Sum  Inputs=|+++
  Sum2 : Sum  Inputs=|-+
  Switch1 : Switch  Threshold=2
  xhat : Outport
  yhat : Outport  Port=2
  wires:
  Gain/1 -> [yhat], yhat/1
  Constant1/1 -> Sum/2
  sigma/1 -> Switch1/2
  Matrix Multiply2/1 -> [A2x]
  Sum/1 -> [sys1]
  Constant4/1 -> Matrix Multiply/1
  Constant2/1 -> Sum1/2
  Integrator1/1 -> [x], xhat/1, Gain/1
  Constant5/1 -> Matrix Multiply2/1
  [x] -> Matrix Multiply2/2, Matrix Multiply/2
  Matrix Multiply/1 -> [A1x]
  Sum1/1 -> [sys2]
  [A2x] -> Sum1/1
  [A1x] -> Sum/1
  [L2y] -> Sum1/3
  [yhat] -> Sum2/1
  y/1 -> Sum2/2
  Sum2/1 -> [ey], Gain2/1, Gain1/1
  Gain2/1 -> [L2y]
  Gain1/1 -> [L1y]
  [L1y] -> Sum/3
  [sys2] -> Switch1/1
  [sys1] -> Switch1/3
  x0/1 -> Integrator1/2
  Switch1/1 -> Integrator1/1  "x"

== system sasControl/Subsystem2/Uncertain Cuk/Subsystem ==
  x : Inport
  u : Inport  Port=2
  Gain : Gain  Gain=B  Multiplication=Matrix(K*u) (u vector)
  Gain1 : Gain  Gain=A  Multiplication=Matrix(K*u) (u vector)
  Gain2 : Gain  Gain=C  Multiplication=Matrix(K*u) (u vector)
  Sum : Sum  Inputs=|++
  xdot : Outport
  y : Outport  Port=2
  wires:
  u/1 -> Gain/1
  x/1 -> Gain2/1, Gain1/1
  Gain1/1 -> Sum/1
  Gain/1 -> Sum/2
  Sum/1 -> xdot/1
  Gain2/1 -> y/1

== system sasControl/Subsystem2/Uncertain Cuk/Subsystem1 ==
  x : Inport
  u : Inport  Port=2
  Gain : Gain  Gain=B  Multiplication=Matrix(K*u) (u vector)
  Gain1 : Gain  Gain=A  Multiplication=Matrix(K*u) (u vector)
  Gain2 : Gain  Gain=C  Multiplication=Matrix(K*u) (u vector)
  Sum : Sum  Inputs=|++
  xdot : Outport
  y : Outport  Port=2
  wires:
  u/1 -> Gain/1
  x/1 -> Gain2/1, Gain1/1
  Gain1/1 -> Sum/1
  Gain/1 -> Sum/2
  Sum/1 -> xdot/1
  Gain2/1 -> y/1
